simulink model "EDS_Simulink_Model_01"  (R2022a)
settings: Solver=VariableStepAuto  StartTime=0.0  StopTime=stop_time  RelTol=1e-3
values from neighbouring files (symbols this model uses):
  a = a/180*pi    [EDS_Script_Model_01.m]    (also in EDS_Script_Model_02.m)
  accel = wheel_radps/accel_time    [EDS_Script_Model_01.m]    (also in EDS_Script_Model_02.m)
  accel_time = 5.33    [EDS_Script_Model_01.m]    (also in EDS_Script_Model_02.m)
  Cx = 0.25    [EDS_Script_Model_01.m]    (also in EDS_Script_Model_02.m)
  d = 1.5    [EDS_Script_Model_01.m]    (also in EDS_Script_Model_02.m)
  density = 1.3    [EDS_Script_Model_01.m]    (also in EDS_Script_Model_02.m)
  Field_DC_voltage_source_1 = 120    [EDS_Script_Model_01.m]
  Field_DC_voltage_source_2 = 120    [EDS_Script_Model_01.m]
  fr = 0.01    [EDS_Script_Model_01.m]    (also in EDS_Script_Model_02.m)
  g = 9.81    [EDS_Script_Model_01.m]    (also in EDS_Script_Model_02.m)
  i_gear = 7.2    [EDS_Script_Model_01.m]    (also in EDS_Script_Model_02.m = 1)
  K_tor_all_1 = 1/2    (= 0.5)    [EDS_Script_Model_01.m]    (also in EDS_Script_Model_02.m)
  K_tor_all_2 = 1/2    (= 0.5)    [EDS_Script_Model_01.m]    (also in EDS_Script_Model_02.m)
  L = 2.5    [EDS_Script_Model_01.m]    (also in EDS_Script_Model_02.m)
  M = 1200    [EDS_Script_Model_01.m]    (also in EDS_Script_Model_02.m)
  n_eff_gear = 0.98    [EDS_Script_Model_01.m]    (also in EDS_Script_Model_02.m = 1)
  output_saturation_lower = -400    [EDS_Script_Model_01.m]
  output_saturation_upper = 400    [EDS_Script_Model_01.m]
  Rw = 0.26    [EDS_Script_Model_01.m]    (also in EDS_Script_Model_02.m)
  S = 1.9    [EDS_Script_Model_01.m]    (also in EDS_Script_Model_02.m)
  steering_angle_1 = steering_angle_1_m(ii)    [EDS_Script_Model_01.m]    (also in EDS_Script_Model_02.m)
  steering_angle_2 = steering_angle_2_m(ii)    [EDS_Script_Model_01.m]    (also in EDS_Script_Model_02.m)
  steering_angle_3 = steering_angle_3_m(ii)    [EDS_Script_Model_01.m]    (also in EDS_Script_Model_02.m)
  steering_angle_4 = steering_angle_4_m(ii)    [EDS_Script_Model_01.m]    (also in EDS_Script_Model_02.m)
  steering_angle_initial = steering_angle_initial_m(ii)    [EDS_Script_Model_01.m]    (also in EDS_Script_Model_02.m)
  time_steering_angle_1 = 8    [EDS_Script_Model_01.m]    (also in EDS_Script_Model_02.m)
  time_steering_angle_2 = 10    [EDS_Script_Model_01.m]    (also in EDS_Script_Model_02.m)
  time_steering_angle_3 = 14    [EDS_Script_Model_01.m]    (also in EDS_Script_Model_02.m)
  time_steering_angle_4 = 18    [EDS_Script_Model_01.m]    (also in EDS_Script_Model_02.m)
undefined symbols (not defined in the file or in its folder): time_w_ref_1, time_w_ref_2, w_ref_1, w_ref_2, w_ref_initial
libraries: spsVoltageMeasurementLib x4, slpidlib x2, spsDCMachineLib x2, spsControlledVoltageSourceLib x2, spsDCVoltageSourceLib x2, spspowerguiLib x1
settings Model: Creator=panos  LastModifiedBy=panos
settings SolverCC: MaxConsecutiveZCs=1500  ZeroCrossAlgorithm=Adaptive
settings DebuggingCC: IgnoredZcDiagnostic=none

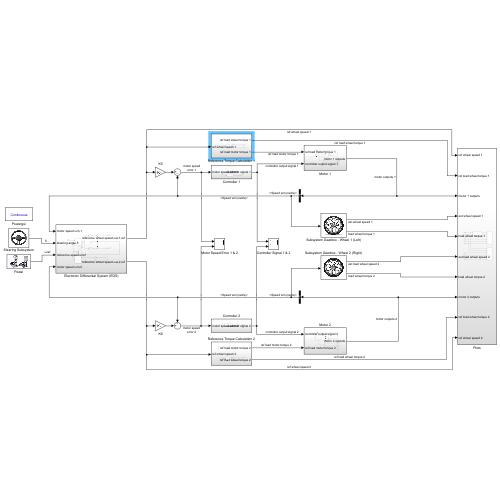
[thumbnail: Simulink's stored preview of the top-level diagram]
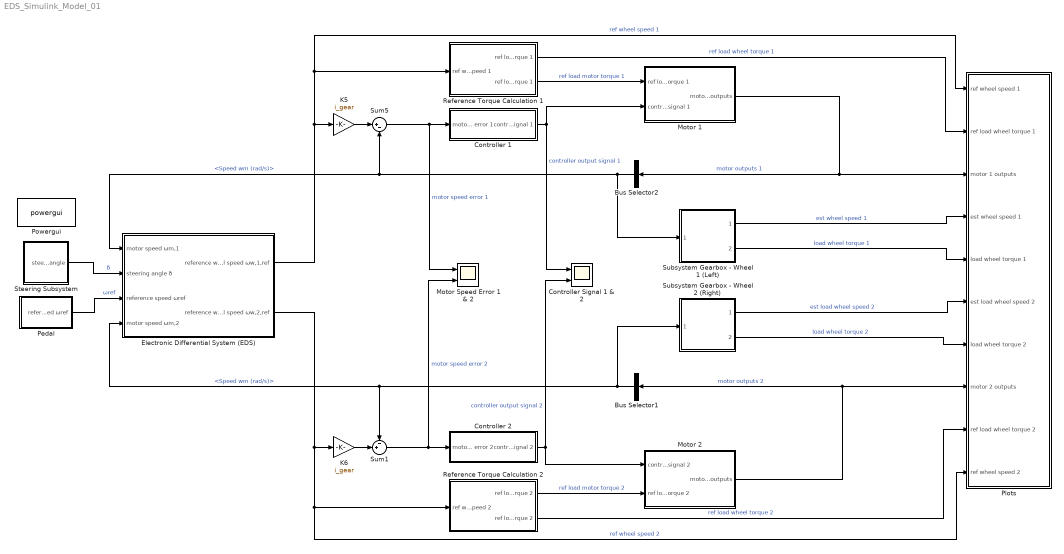
== system EDS_Simulink_Model_01 ==
  Bus Selector1 : BusSelector  OutputSignals=Speed wm (rad/s)
  Bus Selector2 : BusSelector  OutputSignals=Speed wm (rad/s)
  Controller 1 : Subsystem
  Controller 2 : Subsystem
  Controller Signal 1 & 2 : Scope  NumInputPorts=2
  Electronic Differential System (EDS) : Subsystem
  K5 : Gain  Gain=i_gear
  K6 : Gain  Gain=i_gear
  Motor 1 : Subsystem
  Motor 2 : Subsystem
  Motor Speed Error 1 & 2 : Scope  NumInputPorts=2
  Pedal : Subsystem
      mask Display: image('pedal.jpg'); % Use "Edit Image" on toolstrip to change.
  Plots : Subsystem
  Powergui : spspowerguiLib/powergui  Priority=1  SimulationMode=Continuous  SampleTime=50e-6  frequency=60  Iterations=50  frequencyindice=0  Pbase=100e6  ErrMax=1e-4  UnitsV=kV  UnitsW=MW  buscounter=0  FunctionMessages=off  echomessages=off  EnableUseOfTLC=off  CurrentSourceSwitches=off  DisableSnubberDevices=off  DisableRonSwitches=off  DisableVfSwitches=off  DisplayEquations=off  AutomaticDiscreteSolvers=off  SolverType=Tustin/Backward Euler (TBE)  Interpol=off  ExternalGateDelay=off  methode=off  Ts=100  x0status=blocks  SPID=on  SwTol=0  HookPort=off  NonlinearTolerance=1e-4  nMaxIteration=100  ContinueOnMaxIteration=off  RestoreLinks=warning  ResistiveCurrentMeasurement=off  Frange=[0:2:500]  Ylog=off  Xlog=on  ShowGrid=off  save=off  variable=ZData  structure=0  ZoomFFT=off  StartTime=0.0  cycles=1  DisplayStyle=1  fundamental=60  FreqAxis=off  MaxFrequency=1000  frequencyindicesteady=1  RmsSteady=1  display=off
  Reference Torque Calculation 1 : Subsystem
  Reference Torque Calculation 2 : Subsystem
  Steering Subsystem : Subsystem
      mask Display: image('steering.jpg'); % Use "Edit Image" on toolstrip to change.
  Subsystem Gearbox - Wheel 1 (Left) : Subsystem
      mask Display: image('C:\Users\panos\OneDrive\Υπολογιστής\Desktop\Master_Thesis\electronic differential system (EDS)\PHOTO\wheel.jpg'); % Use "Edit Image" on toolstrip to change.
  Subsystem Gearbox - Wheel 2 (Right) : Subsystem
      mask Display: image('C:\Users\panos\OneDrive\Υπολογιστής\Desktop\Master_Thesis\electronic differential system (EDS)\PHOTO\wheel.jpg'); % Use "Edit Image" on toolstrip to change.
  Sum1 : Sum  Inputs=-+|
  Sum5 : Sum  Inputs=|+-
  wires:
  Sum1/1 -> Controller 2/1(motor speed error 2), Motor Speed Error 1 & 2/2  "motor speed error 2"
  Bus Selector1/1 -> Electronic Differential System (EDS)/4(motor speed ωm,2), Sum1/1, Subsystem Gearbox - Wheel 2 (Right)/1(motor speed 2)  "<Speed wm (rad/s)>"
  Sum5/1 -> Controller 1/1(motor speed error 1), Motor Speed Error 1 & 2/1  "motor speed error 1"
  Bus Selector2/1 -> Electronic Differential System (EDS)/1(motor speed ωm,1), Sum5/2, Subsystem Gearbox - Wheel 1 (Left)/1(motor speed 1)  "<Speed wm (rad/s)>"
  Electronic Differential System (EDS)/1("reference wheel speed ωw,1,ref ") -> Plots/1(ref wheel speed 1), Reference Torque Calculation 1/1(ref wheel speed 1), K5/1  "ref wheel speed 1"
  Electronic Differential System (EDS)/2("reference wheel speed ωw,2,ref ") -> Plots/10(ref wheel speed 2), Reference Torque Calculation 2/1(ref wheel speed 2), K6/1  "ref wheel speed 2"
  Motor 1/1(motor 1 outputs) -> Bus Selector2/1, Plots/3(motor 1 outputs)  "motor outputs 1"
  Subsystem Gearbox - Wheel 2 (Right)/1(wheel speed 2) -> Plots/6(est load wheel speed 2)  "est load wheel speed 2"
  Subsystem Gearbox - Wheel 2 (Right)/2(wheel torque 2) -> Plots/7(load wheel torque 2)  "load wheel torque 2"
  Motor 2/1(motor 2 outputs) -> Plots/8(motor 2 outputs), Bus Selector1/1  "motor outputs 2"
  Steering Subsystem/1(steering angle) -> Electronic Differential System (EDS)/2(steering angle δ)  "δ"
  Pedal/1(reference speed ωref) -> Electronic Differential System (EDS)/3(reference speed ωref)  "ωref"
  Reference Torque Calculation 1/2(ref load motor torque 1) -> Motor 1/1(ref load motor torque 1)  "ref load motor torque 1"
  Reference Torque Calculation 1/1(ref load wheel torque 1) -> Plots/2(ref load wheel torque 1)  "ref load wheel torque 1"
  Reference Torque Calculation 2/1(ref load motor torque 2) -> Motor 2/2(ref load motor torque 2)  "ref load motor torque 2"
  Reference Torque Calculation 2/2(ref load wheel torque 2) -> Plots/9(ref load wheel torque 2)  "ref load wheel torque 2"
  Subsystem Gearbox - Wheel 1 (Left)/1(wheel speed 1) -> Plots/4(est wheel speed 1)  "est wheel speed 1"
  Subsystem Gearbox - Wheel 1 (Left)/2(wheel torque 1) -> Plots/5(load wheel torque 1)  "load wheel torque 1"
  K5/1 -> Sum5/1
  K6/1 -> Sum1/2
  Controller 2/1(controller signal 2) -> Controller Signal 1 & 2/2, Motor 2/1(controller output signal 2)  "controller output signal 2"
  Controller 1/1(controller signal 1) -> Controller Signal 1 & 2/1, Motor 1/2(controller output signal 1)  "controller output signal 1"

== system EDS_Simulink_Model_01/Controller 1 ==
  motor speed error 1 : Inport
  "PID " : Subsystem  Commented=on
  PID Controller 1 : slpidlib/PID Controller  Controller=PID  Form=Parallel  TimeDomain=Continuous-time  UseExternalTs=off  SampleTime=-1  IntegratorMethod=Forward Euler  FilterMethod=Forward Euler  ControllerParametersSource=internal  P=5.69713152607283  I=206.821956484623  UseKiTs=off  D=0.0350331064563485  N=22856.5595208321  UseFilter=on  TunerSelectOption=Transfer Function Based (PID Tuner App)  InitialConditionSource=internal  InitialConditionForIntegrator=0  InitialConditionForFilter=0  DifferentiatorICPrevScaledInput=0  ExternalReset=none  TrackingMode=off  Kt=1  LimitOutput=on  SatLimitsSource=internal  UpperSaturationLimit=output_saturation_upper  LowerSaturationLimit=output_saturation_lower  LinearizeAsGain=on  AntiWindupMode=back-calculation  Kb=1  POutMin=[]  POutMax=[]  IOutMin=[]  IOutMax=[]  DOutMin=[]  DOutMax=[]  NOutMin=[]  NOutMax=[]  SumOutMin=[]  SumOutMax=[]  SaturationOutMin=[]  SaturationOutMax=[]  PParamMin=[]  PParamMax=[]  IParamMin=[]  IParamMax=[]  DParamMin=[]  DParamMax=[]  NParamMin=[]  NParamMax=[]  KbParamMin=[]  KbParamMax=[]  KtParamMin=[]  KtParamMax=[]  KbOutMin=[]  KbOutMax=[]  KtOutMin=[]  KtOutMax=[]  IntegratorOutMin=[]  IntegratorOutMax=[]  FilterOutMin=[]  FilterOutMax=[]  SumI1OutMin=[]  SumI1OutMax=[]  SumI2OutMin=[]  SumI2OutMax=[]  SumI3OutMin=[]  SumI3OutMax=[]  SumI4OutMin=[]  SumI4OutMax=[]  SumDOutMin=[]  SumDOutMax=[]  DifferentiatorOutMin=[]  DifferentiatorOutMax=[]  FilterDiffOutCoefMin=[]  FilterDiffOutCoefMax=[]  ReciprocalOutMin=[]  ReciprocalOutMax=[]  SumDenOutMin=[]  SumDenOutMax=[]  SumNumOutMin=[]  SumNumOutMax=[]  DivideOutMin=[]  DivideOutMax=[]  UdiffTsProdOutMin=[]  UdiffTsProdOutMax=[]  NTsProdOutMin=[]  NTsProdOutMax=[]  UintegralTsProdOutMin=[]  UintegralTsProdOutMax=[]  UngainTsProdOutMin=[]  UngainTsProdOutMax=[]  IntegratorContinuousStateAttributes=''  IntegratorStateMustResolveToSignalObject=off  IntegratorRTWStateStorageClass=Auto  FilterContinuousStateAttributes=''  FilterStateMustResolveToSignalObject=off  FilterRTWStateStorageClass=Auto  ParallelPVariant=InternalParameters  IdealPVariant=Disabled  IVariant=InternalParameters  DVariant=InternalParameters  IntegratorVariant=Continuous  SatVariant=Enabled  AWVariant=BackCalculation  PCopyVariant=Disabled  TRVariant=Disabled  FdbkBlocksVariant=Forward  IdealPFdbkVariant=Disabled  SatFdbkVariant=Disabled  DerivativeFilterVariant=ContFilter  NVariant=InternalParameters  NCopyVariant=Disabled  FilterICVariant=InternalICsFilter  IntegratorICVariant=InternalICs  ExternalResetVariant=Disabled  TRSumVariant=Passthrough  SumFdbkVariant=Disabled  SumVariant=Sum_PID  TsampFilterVariant=InternalTs  TsampNgainVariant=Passthrough  TsampIntegralVariant=Passthrough  ExternalSaturationOutDataTypeStr=Inherit: Same as second input  aMode=0
  controller signal 1 : Outport
  wires:
  PID Controller 1/1 -> controller signal 1/1  "controller output signal 1"
  motor speed error 1/1 -> PID Controller 1/1  "ω,er,1"

== system EDS_Simulink_Model_01/Controller 2 ==
  motor speed error 2 : Inport
  PID Controller 2 : slpidlib/PID Controller  Controller=PID  Form=Parallel  TimeDomain=Continuous-time  UseExternalTs=off  SampleTime=-1  IntegratorMethod=Forward Euler  FilterMethod=Forward Euler  ControllerParametersSource=internal  P=5.69713152607283  I=206.821956484623  UseKiTs=off  D=0.0350331064563485  N=22856.5595208321  UseFilter=on  TunerSelectOption=Transfer Function Based (PID Tuner App)  InitialConditionSource=internal  InitialConditionForIntegrator=0  InitialConditionForFilter=0  DifferentiatorICPrevScaledInput=0  ExternalReset=none  TrackingMode=off  Kt=1  LimitOutput=on  SatLimitsSource=internal  UpperSaturationLimit=output_saturation_upper  LowerSaturationLimit=output_saturation_lower  LinearizeAsGain=on  AntiWindupMode=back-calculation  Kb=1  POutMin=[]  POutMax=[]  IOutMin=[]  IOutMax=[]  DOutMin=[]  DOutMax=[]  NOutMin=[]  NOutMax=[]  SumOutMin=[]  SumOutMax=[]  SaturationOutMin=[]  SaturationOutMax=[]  PParamMin=[]  PParamMax=[]  IParamMin=[]  IParamMax=[]  DParamMin=[]  DParamMax=[]  NParamMin=[]  NParamMax=[]  KbParamMin=[]  KbParamMax=[]  KtParamMin=[]  KtParamMax=[]  KbOutMin=[]  KbOutMax=[]  KtOutMin=[]  KtOutMax=[]  IntegratorOutMin=[]  IntegratorOutMax=[]  FilterOutMin=[]  FilterOutMax=[]  SumI1OutMin=[]  SumI1OutMax=[]  SumI2OutMin=[]  SumI2OutMax=[]  SumI3OutMin=[]  SumI3OutMax=[]  SumI4OutMin=[]  SumI4OutMax=[]  SumDOutMin=[]  SumDOutMax=[]  DifferentiatorOutMin=[]  DifferentiatorOutMax=[]  FilterDiffOutCoefMin=[]  FilterDiffOutCoefMax=[]  ReciprocalOutMin=[]  ReciprocalOutMax=[]  SumDenOutMin=[]  SumDenOutMax=[]  SumNumOutMin=[]  SumNumOutMax=[]  DivideOutMin=[]  DivideOutMax=[]  UdiffTsProdOutMin=[]  UdiffTsProdOutMax=[]  NTsProdOutMin=[]  NTsProdOutMax=[]  UintegralTsProdOutMin=[]  UintegralTsProdOutMax=[]  UngainTsProdOutMin=[]  UngainTsProdOutMax=[]  IntegratorContinuousStateAttributes=''  IntegratorStateMustResolveToSignalObject=off  IntegratorRTWStateStorageClass=Auto  FilterContinuousStateAttributes=''  FilterStateMustResolveToSignalObject=off  FilterRTWStateStorageClass=Auto  ParallelPVariant=InternalParameters  IdealPVariant=Disabled  IVariant=InternalParameters  DVariant=InternalParameters  IntegratorVariant=Continuous  SatVariant=Enabled  AWVariant=BackCalculation  PCopyVariant=Disabled  TRVariant=Disabled  FdbkBlocksVariant=Forward  IdealPFdbkVariant=Disabled  SatFdbkVariant=Disabled  DerivativeFilterVariant=ContFilter  NVariant=InternalParameters  NCopyVariant=Disabled  FilterICVariant=InternalICsFilter  IntegratorICVariant=InternalICs  ExternalResetVariant=Disabled  TRSumVariant=Passthrough  SumFdbkVariant=Disabled  SumVariant=Sum_PID  TsampFilterVariant=InternalTs  TsampNgainVariant=Passthrough  TsampIntegralVariant=Passthrough  ExternalSaturationOutDataTypeStr=Inherit: Same as second input  aMode=0
  controller signal 2 : Outport
  wires:
  PID Controller 2/1 -> controller signal 2/1  "controller output signal 2"
  motor speed error 2/1 -> PID Controller 2/1  "ω,er,2"

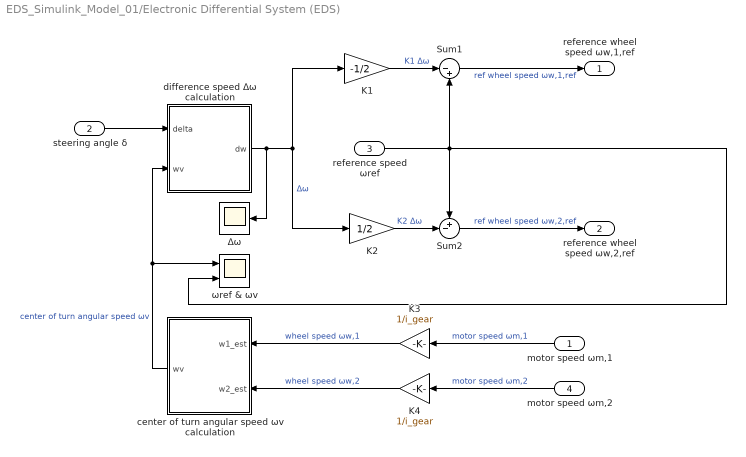
== system EDS_Simulink_Model_01/Electronic Differential System (EDS) ==
  motor speed ωm,1 : Inport
  steering angle δ : Inport  Port=2
  reference speed ωref : Inport  Port=3
  motor speed ωm,2 : Inport  Port=4
  K1 : Gain  Gain=-1/2
  K2 : Gain  Gain=1/2
  K3 : Gain  Gain=1/i_gear
  K4 : Gain  Gain=1/i_gear
  Sum1 : Sum  Inputs=|-+
  Sum2 : Sum  Inputs=+-|
  center of turn angular speed ωv calculation : MATLAB Function  TreatAsAtomicUnit=on
  difference speed Δω calculation : MATLAB Function  TreatAsAtomicUnit=on
  Δω : Scope
  ωref & ωv : Scope  NumInputPorts=2
  "reference wheel speed ωw,1,ref " : Outport
  "reference wheel speed ωw,2,ref " : Outport  Port=2
  wires:
  motor speed ωm,1/1 -> K3/1  "motor speed ωm,1"
  reference speed ωref/1 -> Sum2/1, ωref & ωv/2, Sum1/2
  motor speed ωm,2/1 -> K4/1  "motor speed ωm,2"
  K2/1 -> Sum2/2  "Κ2 Δω"
  K1/1 -> Sum1/1  "Κ1 Δω"
  Sum2/1 -> "reference wheel speed ωw,2,ref "/1  "ref wheel speed ωw,2,ref"
  center of turn angular speed ωv calculation/1(wv) -> difference speed Δω calculation/2(wv), ωref & ωv/1  "center of turn angular speed ωv"
  difference speed Δω calculation/1(dw) -> Δω/1, K2/1, K1/1  "Δω"
  steering angle δ/1 -> difference speed Δω calculation/1(delta)
  K3/1 -> center of turn angular speed ωv calculation/1(w1_est)  "wheel speed ωw,1"
  Sum1/1 -> "reference wheel speed ωw,1,ref "/1  "ref wheel speed ωw,1,ref"
  K4/1 -> center of turn angular speed ωv calculation/2(w2_est)  "wheel speed ωw,2"

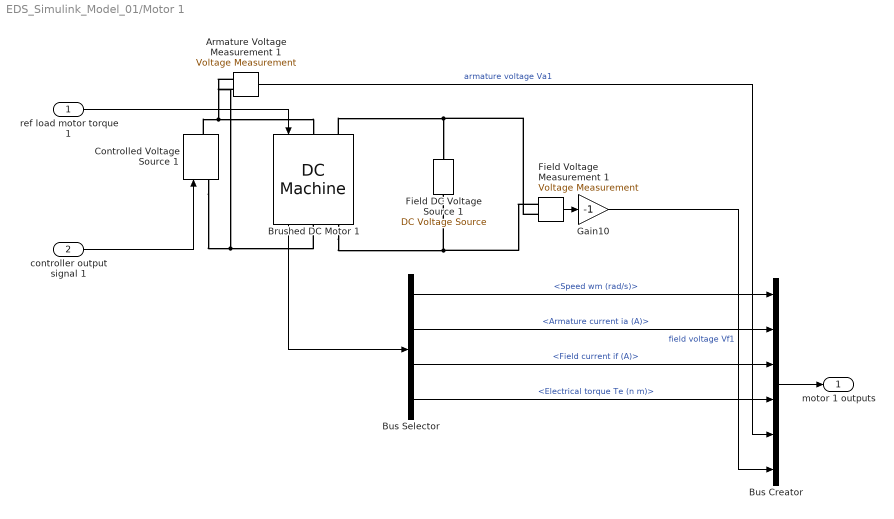
== system EDS_Simulink_Model_01/Motor 1 ==
  ref load motor torque 1 : Inport
  controller output signal 1 : Inport  Port=2
  Armature Voltage Measurement 1 : spsVoltageMeasurementLib/Voltage Measurement  PhasorSimulation=off  OutputType=Complex  PSBequivalent=0
  Brushed DC Motor 1 : spsDCMachineLib/DC Machine  PresetModel=12: 50HP 240V 1750RPM Field:300V  MechanicalLoad=Torque TL  FieldType=Wound  ShowDetailedParameters=on  MeasurementBus=off  RLa=[0.1113 0.001558]  RLf=[84.91 13.39]  Laf=0.3406  MachineConstant=Torque constant (N.m/A)  Ke=1.8  Kt=1.8  J=0.2053  Bm=0.007032  Tf=5.282  w0=Initial_motor_speed  Ifinit=1.41326109998822  TsPowergui=0  TsBlock=-1
  Bus Creator : BusCreator  Inputs=6
  Bus Selector : BusSelector  OutputSignals=Speed wm (rad/s),Armature current ia (A),Field current if (A),Electrical torque Te (n m)
  Controlled Voltage Source 1 : spsControlledVoltageSourceLib/Controlled Voltage Source  Initialize=on  Source_Type=DC  Amplitude=0  Phase=0  Frequency=0  Measurements=Voltage
  Field DC Voltage Source 1 : spsDCVoltageSourceLib/DC Voltage Source  Amplitude=Field_DC_voltage_source_1  Measurements=Voltage
  Field Voltage Measurement 1 : spsVoltageMeasurementLib/Voltage Measurement  PhasorSimulation=off  OutputType=Complex  PSBequivalent=0
  Gain10 : Gain  Gain=-1
  motor 1 outputs : Outport
  wires:
  Field Voltage Measurement 1/1 -> Gain10/1
  ref load motor torque 1/1 -> Brushed DC Motor 1/1
  controller output signal 1/1 -> Controlled Voltage Source 1/1
  Armature Voltage Measurement 1/1 -> Bus Creator/5  "armature voltage Va1"
  Bus Creator/1 -> motor 1 outputs/1
  Brushed DC Motor 1/1 -> Bus Selector/1
  Bus Selector/1 -> Bus Creator/1  "<Speed wm (rad/s)>"
  Bus Selector/2 -> Bus Creator/2  "<Armature current ia (A)>"
  Bus Selector/3 -> Bus Creator/3  "<Field current if (A)>"
  Bus Selector/4 -> Bus Creator/4  "<Electrical torque Te (n m)>"
  Gain10/1 -> Bus Creator/6  "field voltage Vf1"
  connections:
  Field Voltage Measurement 1/LConn2 -- Field DC Voltage Source 1/RConn1 -- Brushed DC Motor 1/LConn2
  Controlled Voltage Source 1/RConn1 -- Armature Voltage Measurement 1/LConn1 -- Brushed DC Motor 1/LConn1
  Brushed DC Motor 1/RConn2 -- Field DC Voltage Source 1/LConn1 -- Field Voltage Measurement 1/LConn1
  Controlled Voltage Source 1/LConn1 -- Brushed DC Motor 1/RConn1 -- Armature Voltage Measurement 1/LConn2

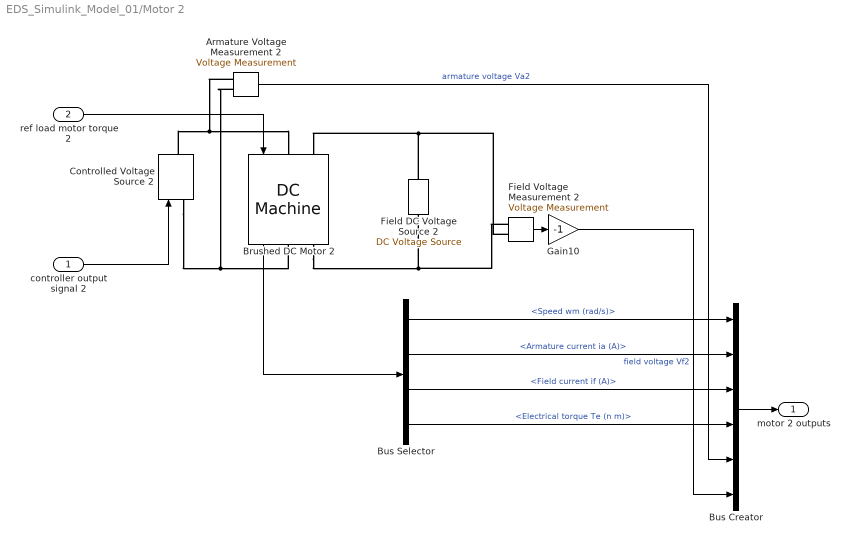
== system EDS_Simulink_Model_01/Motor 2 ==
  controller output signal 2 : Inport
  ref load motor torque 2 : Inport  Port=2
  Armature Voltage Measurement 2 : spsVoltageMeasurementLib/Voltage Measurement  PhasorSimulation=off  OutputType=Complex  PSBequivalent=0
  "Brushed DC Motor 2 " : spsDCMachineLib/DC Machine  PresetModel=12: 50HP 240V 1750RPM Field:300V  MechanicalLoad=Torque TL  FieldType=Wound  ShowDetailedParameters=on  MeasurementBus=off  RLa=[0.1113 0.001558]  RLf=[84.91 13.39]  Laf=0.3406  MachineConstant=Torque constant (N.m/A)  Ke=1.8  Kt=1.8  J=0.2053  Bm=0.007032  Tf=5.282  w0=Initial_motor_speed  Ifinit=1.41326109998822  TsPowergui=0  TsBlock=-1
  Bus Creator : BusCreator  Inputs=6
  Bus Selector : BusSelector  OutputSignals=Speed wm (rad/s),Armature current ia (A),Field current if (A),Electrical torque Te (n m)
  Controlled Voltage Source 2 : spsControlledVoltageSourceLib/Controlled Voltage Source  Initialize=on  Source_Type=DC  Amplitude=0  Phase=0  Frequency=0  Measurements=Voltage
  Field DC Voltage Source 2 : spsDCVoltageSourceLib/DC Voltage Source  Amplitude=Field_DC_voltage_source_2  Measurements=None
  Field Voltage Measurement 2 : spsVoltageMeasurementLib/Voltage Measurement  PhasorSimulation=off  OutputType=Complex  PSBequivalent=0
  Gain10 : Gain  Gain=-1
  motor 2 outputs : Outport
  wires:
  controller output signal 2/1 -> Controlled Voltage Source 2/1
  ref load motor torque 2/1 -> "Brushed DC Motor 2 "/1
  "Brushed DC Motor 2 "/1 -> Bus Selector/1
  Bus Selector/1 -> Bus Creator/1  "<Speed wm (rad/s)>"
  Armature Voltage Measurement 2/1 -> Bus Creator/5  "armature voltage Va2"
  Bus Creator/1 -> motor 2 outputs/1
  Bus Selector/3 -> Bus Creator/3  "<Field current if (A)>"
  Bus Selector/4 -> Bus Creator/4  "<Electrical torque Te (n m)>"
  Field Voltage Measurement 2/1 -> Gain10/1
  Bus Selector/2 -> Bus Creator/2  "<Armature current ia (A)>"
  Gain10/1 -> Bus Creator/6  "field voltage Vf2"
  connections:
  Controlled Voltage Source 2/LConn1 -- "Brushed DC Motor 2 "/RConn1 -- Armature Voltage Measurement 2/LConn2
  Controlled Voltage Source 2/RConn1 -- Armature Voltage Measurement 2/LConn1 -- "Brushed DC Motor 2 "/LConn1
  "Brushed DC Motor 2 "/RConn2 -- Field DC Voltage Source 2/LConn1 -- Field Voltage Measurement 2/LConn1
  Field DC Voltage Source 2/RConn1 -- Field Voltage Measurement 2/LConn2 -- "Brushed DC Motor 2 "/LConn2

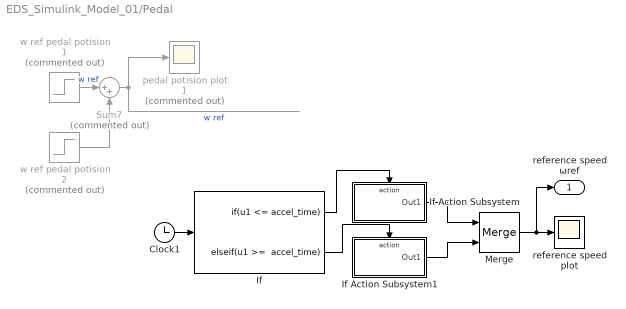
== system EDS_Simulink_Model_01/Pedal ==
  Clock1 : Clock
  If : If  IfExpression=u1 <= accel_time  ElseIfExpressions="u1 >=  accel_time"  ShowElse=off  ZeroCross=off
  If Action Subsystem : Subsystem  TreatAsAtomicUnit=on
  If Action Subsystem1 : Subsystem  TreatAsAtomicUnit=on
  Merge : Merge
  Sum7 : Sum  Commented=on  Inputs=|++
  pedal potision plot 1 : Scope  Commented=on
  reference speed plot : Scope
  w ref pedal potision 1 : Step  Commented=on  Time=time_w_ref_1  Before=w_ref_initial  After=w_ref_1  SampleTime=0
  w ref pedal potision 2 : Step  Commented=on  Time=time_w_ref_2  After=-w_ref_1+w_ref_2  SampleTime=0
  reference speed ωref : Outport
  wires:
  w ref pedal potision 2/1 -> Sum7/2
  w ref pedal potision 1/1 -> Sum7/1  "w ref"
  Sum7/1 -> pedal potision plot 1/1  "w ref"
  Clock1/1 -> If/1
  If/1 -> If Action Subsystem/Action
  If/2 -> If Action Subsystem1/Action
  If Action Subsystem/1(Out1) -> Merge/1
  If Action Subsystem1/1(Out1) -> Merge/2
  Merge/1 -> reference speed plot/1, reference speed ωref/1

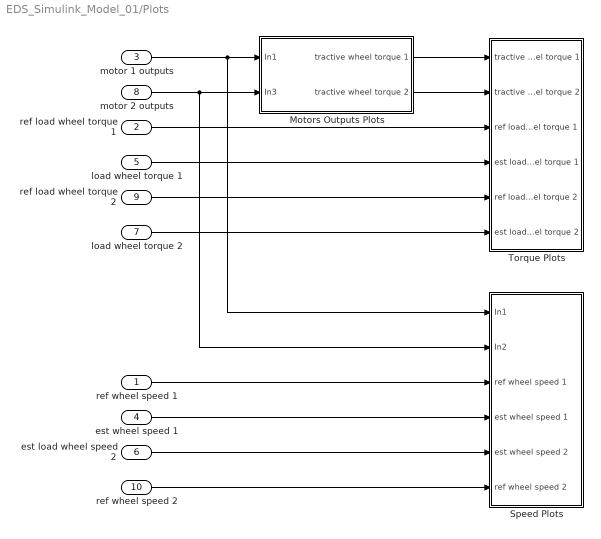
== system EDS_Simulink_Model_01/Plots ==
  ref wheel speed 1 : Inport
  ref load wheel torque 1 : Inport  Port=2
  motor 1 outputs : Inport  Port=3
  est wheel speed 1 : Inport  Port=4
  load wheel torque 1 : Inport  Port=5
  est load wheel speed 2 : Inport  Port=6
  load wheel torque 2 : Inport  Port=7
  motor 2 outputs : Inport  Port=8
  ref load wheel torque 2 : Inport  Port=9
  ref wheel speed 2 : Inport  Port=10
  Motors Outputs Plots : Subsystem
  Speed Plots : Subsystem
  Torque Plots : Subsystem
  wires:
  ref load wheel torque 1/1 -> Torque Plots/3(ref load wheel torque 1)
  Motors Outputs Plots/1(tractive wheel torque 1) -> Torque Plots/1(tractive wheel torque 1)
  Motors Outputs Plots/2(tractive wheel torque 2) -> Torque Plots/2(tractive wheel torque 2)
  load wheel torque 2/1 -> Torque Plots/6(est load wheel torque 2)
  ref load wheel torque 2/1 -> Torque Plots/5(ref load wheel torque 2)
  load wheel torque 1/1 -> Torque Plots/4(est load wheel torque 1)
  motor 2 outputs/1 -> Speed Plots/2(In2), Motors Outputs Plots/2(In3)
  motor 1 outputs/1 -> Speed Plots/1(In1), Motors Outputs Plots/1(In1)
  ref wheel speed 1/1 -> Speed Plots/3(ref wheel speed 1)
  est wheel speed 1/1 -> Speed Plots/4(est wheel speed 1)
  est load wheel speed 2/1 -> Speed Plots/5(est wheel speed 2)
  ref wheel speed 2/1 -> Speed Plots/6(ref wheel speed 2)

== system EDS_Simulink_Model_01/Reference Torque Calculation 1 ==
  ref wheel speed 1 : Inport
  K7 : Gain  Gain=1/(n_eff_gear*i_gear)
  Load Wheel Torque Calculation 1 : MATLAB Function  TreatAsAtomicUnit=on
  acceleration 1 rad/s : Step  Time=accel_time  Before=accel  After=0  SampleTime=0
  ref load wheel torque 1 : Outport
  ref load motor torque 1 : Outport  Port=2
  wires:
  Load Wheel Torque Calculation 1/1(Tw1) -> K7/1, ref load wheel torque 1/1  "ref load wheel torque TLw,1,ref"
  K7/1 -> ref load motor torque 1/1  "ref load motor torque TLm,1,ref"
  ref wheel speed 1/1 -> Load Wheel Torque Calculation 1/1(w1)  "ωw,1,ref"
  acceleration 1 rad/s/1 -> Load Wheel Torque Calculation 1/2(j1)

== system EDS_Simulink_Model_01/Reference Torque Calculation 2 ==
  ref wheel speed 2 : Inport
  K8 : Gain  Gain=1/(n_eff_gear*i_gear)
  Load Wheel Torque Calculation 2 : MATLAB Function  TreatAsAtomicUnit=on
  acceleration 2 rad/s : Step  Time=accel_time  Before=accel  After=0  SampleTime=0
  ref load motor torque 2 : Outport
  ref load wheel torque 2 : Outport  Port=2
  wires:
  Load Wheel Torque Calculation 2/1(Tw2) -> ref load wheel torque 2/1, K8/1  "ref load wheel torque TLw,2,ref"
  ref wheel speed 2/1 -> Load Wheel Torque Calculation 2/1(w2)  "ωw,2,ref"
  K8/1 -> ref load motor torque 2/1  "ref load motor torque TLm,2,ref"
  acceleration 2 rad/s/1 -> Load Wheel Torque Calculation 2/2(j2)

== system EDS_Simulink_Model_01/Steering Subsystem ==
  Sum2 : Sum  Inputs=|++++
  steering angle 1 : Step  Time=time_steering_angle_1  Before=steering_angle_initial  After=steering_angle_1  SampleTime=0
  steering angle 2 : Step  Time=time_steering_angle_2  After=-steering_angle_1+steering_angle_2  SampleTime=0
  steering angle 3 : Step  Time=time_steering_angle_3  After=-steering_angle_2+steering_angle_3  SampleTime=0
  steering angle 4 : Step  Time=time_steering_angle_4  After=-steering_angle_3+steering_angle_4  SampleTime=0
  steering angle plot : Scope
  steering angle : Outport
  wires:
  Sum2/1 -> steering angle plot/1, steering angle/1
  steering angle 1/1 -> Sum2/1
  steering angle 2/1 -> Sum2/2
  steering angle 3/1 -> Sum2/3
  steering angle 4/1 -> Sum2/4

== system EDS_Simulink_Model_01/Subsystem Gearbox - Wheel 1 (Left) ==
  motor speed 1 : Inport
  Gearbox 1 : MATLAB Function  TreatAsAtomicUnit=on
  Load Wheel Torque Calculation 1 : MATLAB Function  TreatAsAtomicUnit=on
  acceleration 1 rad/s : Step  Time=accel_time  Before=accel  After=0  SampleTime=0
  wheel speed 1 : Outport
  wheel torque 1 : Outport  Port=2
  wires:
  Gearbox 1/1(w_speed_1) -> Load Wheel Torque Calculation 1/1(w1), wheel speed 1/1  "wheel speed 1"
  Load Wheel Torque Calculation 1/1(Tw1) -> wheel torque 1/1
  motor speed 1/1 -> Gearbox 1/1(m_speed_1)
  acceleration 1 rad/s/1 -> Load Wheel Torque Calculation 1/2(j1)

== system EDS_Simulink_Model_01/Subsystem Gearbox - Wheel 2 (Right) ==
  motor speed 2 : Inport
  Gearbox 2 : MATLAB Function  TreatAsAtomicUnit=on
  Load Wheel Torque Calculation 2 : MATLAB Function  TreatAsAtomicUnit=on
  acceleration 2 rad/s : Step  Time=accel_time  Before=accel  After=0  SampleTime=0
  wheel speed 2 : Outport
  wheel torque 2 : Outport  Port=2
  wires:
  Gearbox 2/1(w_speed_2) -> Load Wheel Torque Calculation 2/1(w2), wheel speed 2/1  "wheel speed 2"
  Load Wheel Torque Calculation 2/1(Tw2) -> wheel torque 2/1
  motor speed 2/1 -> Gearbox 2/1(m_speed_2)
  acceleration 2 rad/s/1 -> Load Wheel Torque Calculation 2/2(j2)

== system EDS_Simulink_Model_01/Controller 1/PID  ==
  In1 : Inport
  Derivative1 : Derivative
  Integrator : Integrator
  Kd (Gain) : Gain
  Ki (Gain) : Gain  Gain=5
  Kp (Gain) : Gain  Gain=5
  Saturation : Saturate  UpperLimit=2  LowerLimit=-2
  Sum1 : Sum  Inputs=+++
  Out1 : Outport
  wires:
  Sum1/1 -> Saturation/1  "v(t)"
  In1/1 -> Derivative1/1, Kp (Gain)/1, Integrator/1
  Derivative1/1 -> Kd (Gain)/1
  Kd (Gain)/1 -> Sum1/3  "v(t)"
  Kp (Gain)/1 -> Sum1/2  "v(t)"
  Integrator/1 -> Ki (Gain)/1
  Ki (Gain)/1 -> Sum1/1
  Saturation/1 -> Out1/1

== system EDS_Simulink_Model_01/Pedal/If Action Subsystem ==
  Action Port : ActionPort  ActionPortLabel=if(u1 <= accel_time)
  Clock : Clock
      settings: Decimation=5
  fun3 : MATLAB Function  TreatAsAtomicUnit=on
  Out1 : Outport
  wires:
  fun3/1(y) -> Out1/1
  Clock/1 -> fun3/1(x)

== system EDS_Simulink_Model_01/Pedal/If Action Subsystem1 ==
  Action Port : ActionPort  ActionPortLabel="elseif(u1 >=  accel_time)"
  fun3 : MATLAB Function  TreatAsAtomicUnit=on
  Out1 : Outport
  wires:
  fun3/1(y) -> Out1/1

== system EDS_Simulink_Model_01/Plots/Motors Outputs Plots ==
  In1 : Inport
  In3 : Inport  Port=2
  Gain8 : Gain  Gain=(i_gear * n_eff_gear)
  Gain9 : Gain  Gain=(i_gear * n_eff_gear)
  Motor Outputs 1 : Subsystem
  Motor Outputs 1&2 : Subsystem
  Motor Outputs 2 : Subsystem
  tractive wheel torque 1 : Outport
  tractive wheel torque 2 : Outport  Port=2
  wires:
  In3/1 -> Motor Outputs 1&2/2(In2), Motor Outputs 2/1(In1)
  In1/1 -> Motor Outputs 1&2/1(In1), Motor Outputs 1/1(In1)
  Gain8/1 -> tractive wheel torque 1/1  "tractive wheel torque 1"
  Motor Outputs 1/1(Output) -> Gain8/1
  Motor Outputs 2/1(Output) -> Gain9/1
  Gain9/1 -> tractive wheel torque 2/1  "tractive wheel torque 2"

== system EDS_Simulink_Model_01/Plots/Speed Plots ==
  In1 : Inport
  In2 : Inport  Port=2
  ref wheel speed 1 : Inport  Port=3
  est wheel speed 1 : Inport  Port=4
  est wheel speed 2 : Inport  Port=5
  ref wheel speed 2 : Inport  Port=6
  Bus Selector1 : BusSelector  OutputSignals=Speed wm (rad/s)
  Bus Selector3 : BusSelector  OutputSignals=Speed wm (rad/s)
  Motor Speed Plots (rad/s) : Subsystem
  Wheel Speed Plots : Subsystem
  wires:
  Bus Selector1/1 -> Motor Speed Plots (rad/s)/2(wm,2)  "<Speed wm (rad/s)>"
  ref wheel speed 1/1 -> Motor Speed Plots (rad/s)/3(ωw,1,ref), Wheel Speed Plots/1(ref wheel speed 1)
  Bus Selector3/1 -> Motor Speed Plots (rad/s)/1(wm,1)  "<Speed wm (rad/s)>"
  ref wheel speed 2/1 -> Motor Speed Plots (rad/s)/4(ωw,2,ref), Wheel Speed Plots/4(ref wheel speed 2)
  est wheel speed 1/1 -> Wheel Speed Plots/2(est wheel speed 1)
  In1/1 -> Bus Selector3/1
  est wheel speed 2/1 -> Wheel Speed Plots/3(est wheel speed 2)
  In2/1 -> Bus Selector1/1

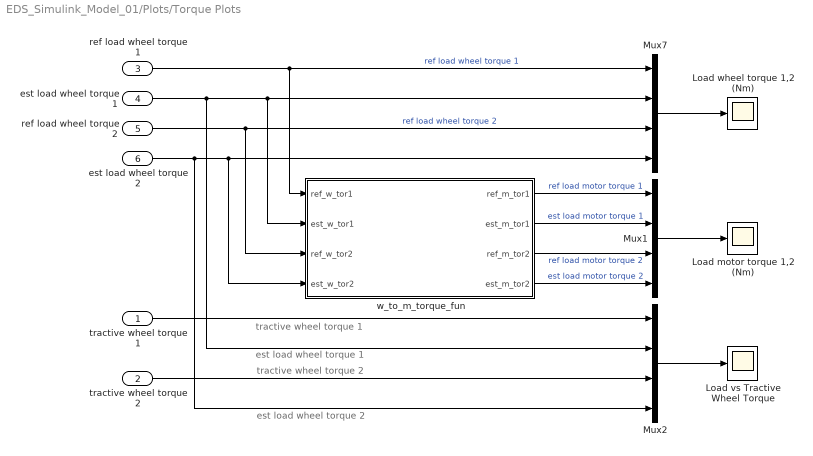
== system EDS_Simulink_Model_01/Plots/Torque Plots ==
  note: est load wheel torque 2
  note: tractive wheel torque 2
  note: tractive wheel torque 1
  note: est load wheel torque 1
  tractive wheel torque 1 : Inport
  tractive wheel torque 2 : Inport  Port=2
  ref load wheel torque 1 : Inport  Port=3
  est load wheel torque 1 : Inport  Port=4
  ref load wheel torque 2 : Inport  Port=5
  est load wheel torque 2 : Inport  Port=6
  Load motor torque 1,2 (Nm) : Scope
  Load vs Tractive Wheel Torque : Scope
  Load wheel torque 1,2 (Nm) : Scope
  Mux1 : Mux
  Mux2 : Mux
  Mux7 : Mux
  w_to_m_torque_fun : MATLAB Function  TreatAsAtomicUnit=on
  wires:
  w_to_m_torque_fun/3(ref_m_tor2) -> Mux1/3  "ref load motor torque 2"
  est load wheel torque 1/1 -> Mux7/2, w_to_m_torque_fun/2(est_w_tor1), Mux2/2
  w_to_m_torque_fun/2(est_m_tor1) -> Mux1/2  "est load motor torque 1"
  ref load wheel torque 2/1 -> w_to_m_torque_fun/3(ref_w_tor2), Mux7/3  "ref load wheel torque 2"
  w_to_m_torque_fun/4(est_m_tor2) -> Mux1/4  "est load motor torque 2"
  est load wheel torque 2/1 -> Mux7/4, w_to_m_torque_fun/4(est_w_tor2), Mux2/4
  w_to_m_torque_fun/1(ref_m_tor1) -> Mux1/1  "ref load motor torque 1"
  ref load wheel torque 1/1 -> w_to_m_torque_fun/1(ref_w_tor1), Mux7/1  "ref load wheel torque 1"
  Mux7/1 -> Load wheel torque 1,2 (Nm)/1
  Mux1/1 -> Load motor torque 1,2 (Nm)/1
  tractive wheel torque 2/1 -> Mux2/3
  tractive wheel torque 1/1 -> Mux2/1
  Mux2/1 -> Load vs Tractive Wheel Torque/1

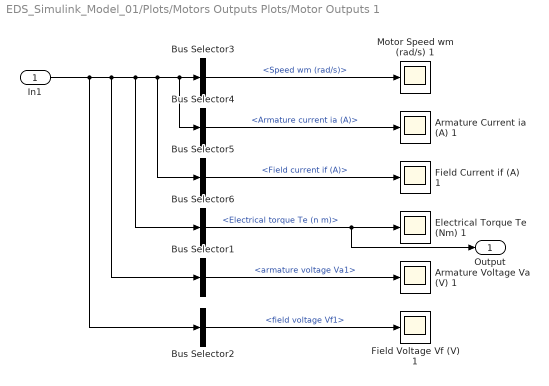
== system EDS_Simulink_Model_01/Plots/Motors Outputs Plots/Motor Outputs 1 ==
  In1 : Inport
  Armature Current ia (A) 1 : Scope
  Armature Voltage Va (V) 1 : Scope
  Bus Selector1 : BusSelector  OutputSignals=armature voltage Va1
  Bus Selector2 : BusSelector  OutputSignals=field voltage Vf1
  Bus Selector3 : BusSelector  OutputSignals=Speed wm (rad/s)
  Bus Selector4 : BusSelector  OutputSignals=Armature current ia (A)
  Bus Selector5 : BusSelector  OutputSignals=Field current if (A)
  Bus Selector6 : BusSelector  OutputSignals=Electrical torque Te (n m)
  Electrical Torque Te (Nm) 1 : Scope
  Field Current if (A) 1 : Scope
  Field Voltage Vf (V) 1 : Scope
  Motor Speed wm (rad/s) 1 : Scope
  Output : Outport
  wires:
  In1/1 -> Bus Selector2/1, Bus Selector1/1, Bus Selector6/1, Bus Selector5/1, Bus Selector4/1, Bus Selector3/1
  Bus Selector5/1 -> Field Current if (A) 1/1  "<Field current if (A)>"
  Bus Selector6/1 -> Electrical Torque Te (Nm) 1/1, Output/1  "<Electrical torque Te (n m)>"
  Bus Selector3/1 -> Motor Speed wm (rad/s) 1/1  "<Speed wm (rad/s)>"
  Bus Selector4/1 -> Armature Current ia (A) 1/1  "<Armature current ia (A)>"
  Bus Selector1/1 -> Armature Voltage Va (V) 1/1  "<armature voltage Va1>"
  Bus Selector2/1 -> Field Voltage Vf (V) 1/1  "<field voltage Vf1>"

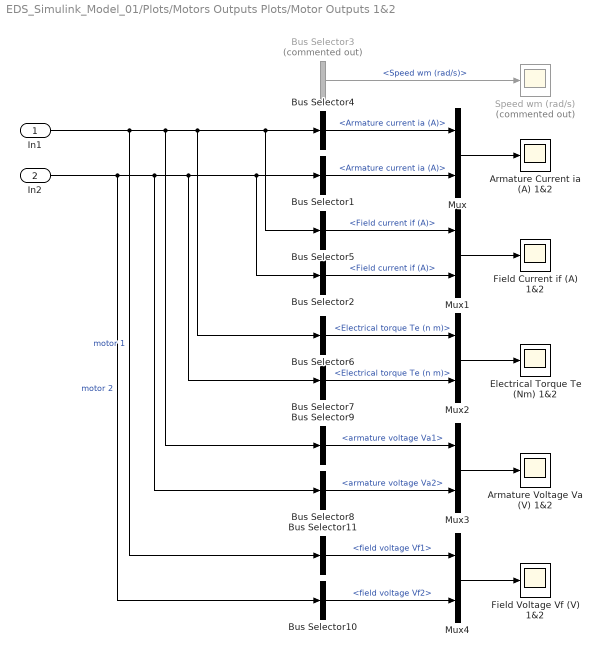
== system EDS_Simulink_Model_01/Plots/Motors Outputs Plots/Motor Outputs 1&2 ==
  In1 : Inport
  In2 : Inport  Port=2
  Armature Current ia (A) 1&2 : Scope
  Armature Voltage Va (V) 1&2 : Scope
  Bus Selector1 : BusSelector  OutputSignals=Armature current ia (A)
  Bus Selector10 : BusSelector  OutputSignals=field voltage Vf2
  Bus Selector11 : BusSelector  OutputSignals=field voltage Vf1
  Bus Selector2 : BusSelector  OutputSignals=Field current if (A)
  Bus Selector3 : BusSelector  Commented=on  OutputSignals=Speed wm (rad/s)
  Bus Selector4 : BusSelector  OutputSignals=Armature current ia (A)
  Bus Selector5 : BusSelector  OutputSignals=Field current if (A)
  Bus Selector6 : BusSelector  OutputSignals=Electrical torque Te (n m)
  Bus Selector7 : BusSelector  OutputSignals=Electrical torque Te (n m)
  Bus Selector8 : BusSelector  OutputSignals=armature voltage Va2
  Bus Selector9 : BusSelector  OutputSignals=armature voltage Va1
  Electrical Torque Te (Nm) 1&2 : Scope
  Field Current if (A) 1&2 : Scope
  Field Voltage Vf (V) 1&2 : Scope
  Mux{,1..4} (5 alike) : Mux  Inputs=2
  Speed wm (rad/s) : Scope  Commented=on
  wires:
  In1/1 -> Bus Selector11/1, Bus Selector9/1, Bus Selector6/1, Bus Selector5/1, Bus Selector4/1  "motor 1"
  Bus Selector3/1 -> Speed wm (rad/s)/1  "<Speed wm (rad/s)>"
  Bus Selector4/1 -> Mux/1  "<Armature current ia (A)>"
  Bus Selector1/1 -> Mux/2  "<Armature current ia (A)>"
  Mux/1 -> Armature Current ia (A) 1&2/1
  Bus Selector2/1 -> Mux1/2  "<Field current if (A)>"
  Bus Selector5/1 -> Mux1/1  "<Field current if (A)>"
  Mux1/1 -> Field Current if (A) 1&2/1
  Bus Selector6/1 -> Mux2/1  "<Electrical torque Te (n m)>"
  Mux2/1 -> Electrical Torque Te (Nm) 1&2/1
  Bus Selector7/1 -> Mux2/2  "<Electrical torque Te (n m)>"
  In2/1 -> Bus Selector10/1, Bus Selector8/1, Bus Selector7/1, Bus Selector2/1, Bus Selector1/1  "motor 2"
  Mux3/1 -> Armature Voltage Va (V) 1&2/1
  Bus Selector9/1 -> Mux3/1  "<armature voltage Va1>"
  Bus Selector8/1 -> Mux3/2  "<armature voltage Va2>"
  Bus Selector11/1 -> Mux4/1  "<field voltage Vf1>"
  Bus Selector10/1 -> Mux4/2  "<field voltage Vf2>"
  Mux4/1 -> Field Voltage Vf (V) 1&2/1

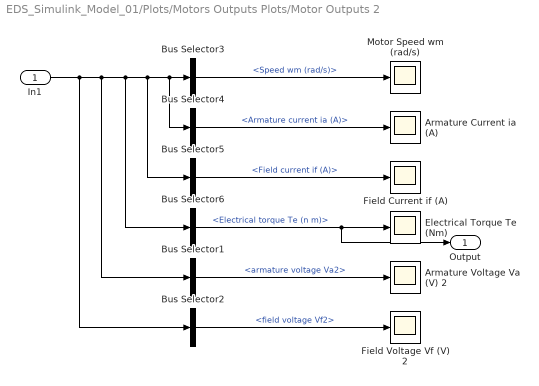
== system EDS_Simulink_Model_01/Plots/Motors Outputs Plots/Motor Outputs 2 ==
  In1 : Inport
  Armature Current ia (A) : Scope
  Armature Voltage Va (V) 2 : Scope
  Bus Selector1 : BusSelector  OutputSignals=armature voltage Va2
  Bus Selector2 : BusSelector  OutputSignals=field voltage Vf2
  Bus Selector3 : BusSelector  OutputSignals=Speed wm (rad/s)
  Bus Selector4 : BusSelector  OutputSignals=Armature current ia (A)
  Bus Selector5 : BusSelector  OutputSignals=Field current if (A)
  Bus Selector6 : BusSelector  OutputSignals=Electrical torque Te (n m)
  Electrical Torque Te (Nm) : Scope
  Field Current if (A) : Scope
  Field Voltage Vf (V) 2 : Scope
  Motor Speed wm (rad/s) : Scope
  Output : Outport
  wires:
  In1/1 -> Bus Selector2/1, Bus Selector1/1, Bus Selector6/1, Bus Selector5/1, Bus Selector4/1, Bus Selector3/1
  Bus Selector5/1 -> Field Current if (A)/1  "<Field current if (A)>"
  Bus Selector6/1 -> Electrical Torque Te (Nm)/1, Output/1  "<Electrical torque Te (n m)>"
  Bus Selector3/1 -> Motor Speed wm (rad/s)/1  "<Speed wm (rad/s)>"
  Bus Selector4/1 -> Armature Current ia (A)/1  "<Armature current ia (A)>"
  Bus Selector1/1 -> Armature Voltage Va (V) 2/1  "<armature voltage Va2>"
  Bus Selector2/1 -> Field Voltage Vf (V) 2/1  "<field voltage Vf2>"

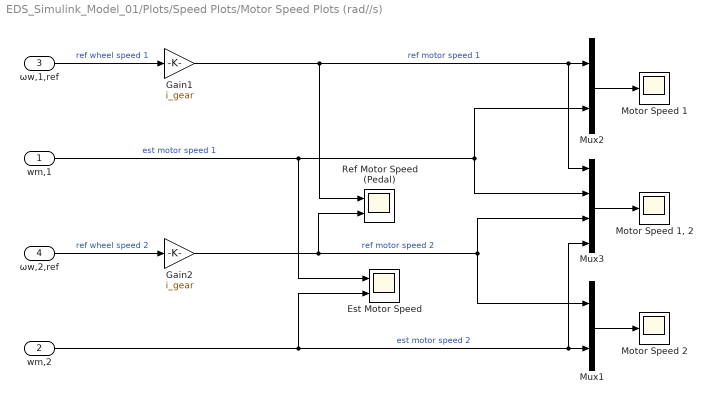
== system EDS_Simulink_Model_01/Plots/Speed Plots/Motor Speed Plots (rad//s) ==
  wm,1 : Inport
  wm,2 : Inport  Port=2
  ωw,1,ref : Inport  Port=3
  ωw,2,ref : Inport  Port=4
  Est Motor Speed : Scope  NumInputPorts=2
  Gain1 : Gain  Gain=i_gear
  Gain2 : Gain  Gain=i_gear
  Motor Speed 1 : Scope
  "Motor Speed 1, 2" : Scope
  Motor Speed 2 : Scope
  Mux1 : Mux  Inputs=2
  Mux2 : Mux  Inputs=2
  Mux3 : Mux
  Ref Motor Speed (Pedal) : Scope  NumInputPorts=2
  wires:
  ωw,2,ref/1 -> Gain2/1  "ref wheel speed 2"
  wm,1/1 -> Mux3/2, Mux2/2, Est Motor Speed/1  "est motor speed 1"
  wm,2/1 -> Est Motor Speed/2, Mux3/4, Mux1/2  "est motor speed 2"
  Mux1/1 -> Motor Speed 2/1
  ωw,1,ref/1 -> Gain1/1  "ref wheel speed 1"
  Mux3/1 -> "Motor Speed 1, 2"/1
  Mux2/1 -> Motor Speed 1/1
  Gain1/1 -> Mux2/1, Mux3/1, Ref Motor Speed (Pedal)/1  "ref motor speed 1"
  Gain2/1 -> Mux1/1, Mux3/3, Ref Motor Speed (Pedal)/2  "ref motor speed 2"

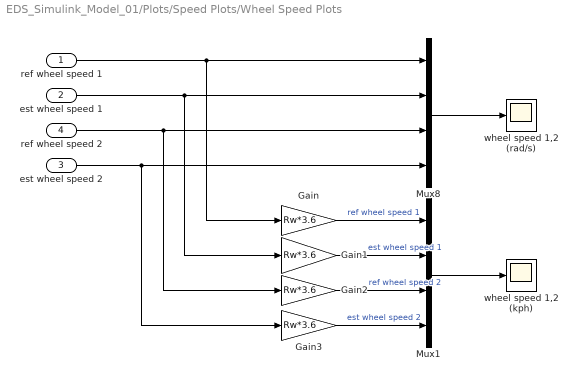
== system EDS_Simulink_Model_01/Plots/Speed Plots/Wheel Speed Plots ==
  ref wheel speed 1 : Inport
  est wheel speed 1 : Inport  Port=2
  est wheel speed 2 : Inport  Port=3
  ref wheel speed 2 : Inport  Port=4
  Gain{,1..3} (4 alike) : Gain  Gain=Rw*3.6
  Mux1 : Mux
  Mux8 : Mux
  wheel speed 1,2 (kph) : Scope
  wheel speed 1,2 (rad/s) : Scope
  wires:
  Mux8/1 -> wheel speed 1,2 (rad/s)/1
  Mux1/1 -> wheel speed 1,2 (kph)/1
  ref wheel speed 1/1 -> Mux8/1, Gain/1
  ref wheel speed 2/1 -> Mux8/3, Gain2/1
  Gain/1 -> Mux1/1  "ref wheel speed 1"
  est wheel speed 1/1 -> Mux8/2, Gain1/1
  Gain1/1 -> Mux1/2  "est wheel speed 1"
  Gain3/1 -> Mux1/4  "est wheel speed 2"
  Gain2/1 -> Mux1/3  "ref wheel speed 2"
  est wheel speed 2/1 -> Mux8/4, Gain3/1

== matlab function EDS_Simulink_Model_01/Electronic Differential System (EDS)/difference speed Δω calculation ==
  data: delta input; wv input; dw output; d parameter; L parameter; pi parameter
function dw = dw_fun(delta, wv, d, L, pi)

% delta : input     : [deg] steering angle
% wv    : input     : [rad/s] vehicle angular speed according to the center of turn
% L     : parameter : [m] wheelbase or distance between two wheels and axes
% d     : parameter : [m] distance between the wheels of the same axle
% dw    : output    : [rad/s] the difference between wheel drive angular speeds

delta = delta * pi/180;          % convert steering angle delta from deg to rad
dw    = - d * tan(delta)/L * wv;

== matlab function EDS_Simulink_Model_01/Subsystem Gearbox - Wheel 1 (Left)/Gearbox 1 ==
  data: m_speed_1 input; w_speed_1 output; i_gear parameter
function w_speed_1  = Gear_fun_1(m_speed_1,i_gear)

% w : wheel
% m : motor
w_speed_1  = m_speed_1 / i_gear;



% function [w_speed_1, w_torque_1] = Gear_fun_1(m_speed_1,m_torque_1,i_gear,n_eff_gear)
% 
% % w : wheel
% % m : motor
% 
% w_torque_1 = m_torque_1 * i_gear * n_eff_gear;
% w_speed_1  = m_speed_1 / i_gear;

== matlab function EDS_Simulink_Model_01/Subsystem Gearbox - Wheel 2 (Right)/Gearbox 2 ==
  data: m_speed_2 input; w_speed_2 output; i_gear parameter
function w_speed_2  = Gear_fun_2(m_speed_2,i_gear)

% w : wheel
% m : motor
w_speed_2  = m_speed_2 / i_gear;

== matlab function EDS_Simulink_Model_01/Subsystem Gearbox - Wheel 1 (Left)/Load Wheel Torque Calculation 1 ==
  data: w1 input; j1 input; Tw1 output; a parameter; fr parameter; Rw parameter; Cx parameter; S parameter; M parameter; density parameter; K_tor_all_1 parameter; g parameter
function Tw1 = Tw1_fun(w1, j1, a, fr, Rw, Cx, S, M, density, K_tor_all_1, g)

% w1          : input     : [rad/s]  Angular speed of drive wheel 1 (left)
% a           : parameter : [deg]    Grade angle of the road
% fr          : parameter : [-]      Vehicle friction coefficient
% Rw          : parameter : [m]      Wheel radius
% M           : parameter : [kg]     Vehicle mass
% S           : parameter : [m^2]    Vehicle frontal area
% density     : parameter : [kg/m^3] Air density
% Cx          : parameter : [-]      Aerodynamic drag coefficient
% g           : parameter : [m/s^2]  Gravitational acceleration 
% K_tor_all_1 : parameter : [-]      Torque allocation in wheel 1
% Tslope      : parameter : [Nm]     Vehicle torque
% Ttire       : parameter : [Nm]     Tire torque
% Taero       : parameter : [Nm]     Aerodynamique torque
% Tw1         : output    : [Nm]     Load torque that wheel 1 have to overcome

Tslope = M*g*sin(a)*Rw;                
Ttire  = M*g*fr*Rw;                       
Taero  = 1/2*density*S*Cx*Rw^3*w1^2;  
Tinertia = M*j1*Rw^2;
Tw1    = K_tor_all_1 * (Tslope + Ttire + Taero + Tinertia);

== matlab function EDS_Simulink_Model_01/Subsystem Gearbox - Wheel 2 (Right)/Load Wheel Torque Calculation 2 ==
  data: w2 input; j2 input; Tw2 output; a parameter; fr parameter; Rw parameter; Cx parameter; S parameter; M parameter; density parameter; K_tor_all_2 parameter; g parameter
function Tw2  = Tw2_fun(w2, j2, a, fr, Rw, Cx, S, M, density, K_tor_all_2, g)

% w2          : input     : [rad/s]  Angular speed of drive wheel 2 (right)
% a           : parameter : [deg]    Grade angle of the road
% fr          : parameter : [-]      Vehicle friction coefficient
% Rw          : parameter : [m]      Wheel radius
% M           : parameter : [kg]     Vehicle mass
% S           : parameter : [m^2]    Vehicle frontal area
% density     : parameter : [kg/m^3] Air density
% Cx          : parameter : [-]      Aerodynamic drag coefficient
% g           : parameter : [m/s^2]  Gravitational acceleration 
% K_tor_all_2 : parameter : [-]      Torque allocation in wheel 2
% Tslope      : parameter : [Nm]     Vehicle torque
% Ttire       : parameter : [Nm]     Tire torque
% Taero       : parameter : [Nm]     Aerodynamique torque
% Tw2         : output    : [Nm]     Load torque that wheel 2 have to overcome

Tslope = M*g*sin(a)*Rw;                 
Ttire  = M*g*fr*Rw;                      
Taero  = 1/2*density*S*Cx*Rw^3*w2^2;  
Tinertia = M*j2*Rw^2;
Tw2    = K_tor_all_2 * (Tslope + Ttire + Taero + Tinertia);

== matlab function EDS_Simulink_Model_01/Plots/Torque Plots/w_to_m_torque_fun ==
  data: ref_w_tor1 input; est_w_tor1 input; ref_w_tor2 input; est_w_tor2 input; ref_m_tor1 output; est_m_tor1 output; ref_m_tor2 output; est_m_tor2 output; i_gear parameter; n_eff_gear parameter
function [ref_m_tor1, est_m_tor1, ref_m_tor2, est_m_tor2] = ...
  w_to_m_torque_fun(ref_w_tor1, est_w_tor1, ref_w_tor2, est_w_tor2, i_gear, n_eff_gear)

% w : wheel
% m : motor

% ref_w_tor1 = ref_m_tor1 * i_gear * n_eff_gear;
ref_m_tor1 = ref_w_tor1 / (i_gear * n_eff_gear);
est_m_tor1 = est_w_tor1 / (i_gear * n_eff_gear);
ref_m_tor2 = ref_w_tor2 / (i_gear * n_eff_gear);
est_m_tor2 = est_w_tor2 / (i_gear * n_eff_gear);

== matlab function EDS_Simulink_Model_01/Pedal/If Action Subsystem/fun3 ==
  data: x input; y output; accel parameter
function y = accel1_fun(x,accel)

y = accel*x;

== matlab function EDS_Simulink_Model_01/Pedal/If Action Subsystem1/fun3 ==
  data: y output; accel parameter; accel_time parameter
function y = accel1_fun(accel, accel_time)

y = accel*accel_time;

== matlab function EDS_Simulink_Model_01/Electronic Differential System (EDS)/center of turn angular speed ωv calculation ==
  data: w1_est input; w2_est input; wv output
function wv = wv_fun(w1_est, w2_est)

% w1_est : input : [rad/s] actual angular speed of drive wheel 1 (left)
% w2_est : input : [rad/s] actual angular speed of drive wheel 2 (right)
% wv     : outpt : [rad/s] vehicle angular speed according to the center of turn

wv = (w1_est + w2_est) / 2;

== matlab function EDS_Simulink_Model_01/Reference Torque Calculation 1/Load Wheel Torque Calculation 1 ==
  data: w1 input; j1 input; Tw1 output; a parameter; fr parameter; Rw parameter; Cx parameter; S parameter; M parameter; density parameter; K_tor_all_1 parameter; g parameter
function Tw1 = Tw1_fun(w1, j1, a, fr, Rw, Cx, S, M, density, K_tor_all_1, g)

% w1          : input     : [rad/s]   Angular speed of drive wheel 1 (left)
% j1          : input     : [rad/s^2] Angular acceleration of drive wheel 1 (left)
% a           : parameter : [deg]     Grade angle of the road
% fr          : parameter : [-]       Vehicle friction coefficient
% Rw          : parameter : [m]       Wheel radius
% M           : parameter : [kg]      Vehicle mass
% S           : parameter : [m^2]     Vehicle frontal area
% density     : parameter : [kg/m^3]  Air density
% Cx          : parameter : [-]       Aerodynamic drag coefficient
% g           : parameter : [m/s^2]   Gravitational acceleration 
% K_tor_all_1 : parameter : [-]       Torque allocation in wheel 1
% Tslope      : parameter : [Nm]      Vehicle torque
% Ttire       : parameter : [Nm]      Tire torque
% Taero       : parameter : [Nm]      Aerodynamique torque
% Tw1         : output    : [Nm]      Load torque that wheel 1 have to overcome

Tslope = M*g*sin(a)*Rw;                
Ttire  = M*g*fr*Rw;                       
Taero  = 1/2*density*S*Cx*Rw^3*w1^2;  
Tinertia = M*j1*Rw^2;
Tw1    = K_tor_all_1 * (Tslope + Ttire + Taero + Tinertia);

== matlab function EDS_Simulink_Model_01/Reference Torque Calculation 2/Load Wheel Torque Calculation 2 ==
  data: w2 input; j2 input; Tw2 output; a parameter; fr parameter; Rw parameter; Cx parameter; S parameter; M parameter; density parameter; K_tor_all_2 parameter; g parameter
function Tw2  = Tw2_fun(w2, j2, a, fr, Rw, Cx, S, M, density, K_tor_all_2, g)

% w2          : input     : [rad/s]   Angular speed of drive wheel 2 (right)
% j2          : input     : [rad/s^2] Angular acceleration of drive wheel 2 (right)
% a           : parameter : [deg]     Grade angle of the road
% fr          : parameter : [-]       Vehicle friction coefficient
% Rw          : parameter : [m]       Wheel radius
% M           : parameter : [kg]      Vehicle mass
% S           : parameter : [m^2]     Vehicle frontal area
% density     : parameter : [kg/m^3]  Air density
% Cx          : parameter : [-]       Aerodynamic drag coefficient
% g           : parameter : [m/s^2]   Gravitational acceleration 
% K_tor_all_2 : parameter : [-]       Torque allocation in wheel 2
% Tslope      : parameter : [Nm]      Vehicle torque
% Ttire       : parameter : [Nm]      Tire torque
% Taero       : parameter : [Nm]      Aerodynamique torque
% Tw2         : output    : [Nm]      Load torque that wheel 2 have to overcome

Tslope = M*g*sin(a)*Rw;                 
Ttire  = M*g*fr*Rw;                      
Taero  = 1/2*density*S*Cx*Rw^3*w2^2;  
Tinertia = M*j2*Rw^2;
Tw2    = K_tor_all_2 * (Tslope + Ttire + Taero + Tinertia);
